simulink model "System_model"  (R2024b)
settings: Solver=ode1  StartTime=0.0  StopTime=12*3600  FixedStep=3600  RelTol=1e-3
values from neighbouring files (symbols this model uses):
  c = c_joule/3600    (= 1.16666666667)    [Dynamic.m]    (also in flat_plate_DHW.m = 4200)
  Ta = (Tmax+Tmin)/2 +(Tmax-Tmin)/2*cos(2*pi/24*(time_sun-tmax))    [Dynamic.m]    (also in flat_plate_DHW.m = (Ta_min+Ta_max)/2 + (-Ta_min+Ta_max)/2*cos(2*pi/24*(t-12)))
  time = (0:60*24)'    [Dynamic.m]
  Ts0 = out.Ts(end)    [parametric_analysis.m]
undefined symbols (not defined in the file or in its folder): dQd, dQr, hA, M
settings Model: Creator=giacm  LastModifiedBy=Andrea
settings DataIOCC: ReturnWorkspaceOutputs=off
settings RTWCC: GPUComputeCapability=3.5

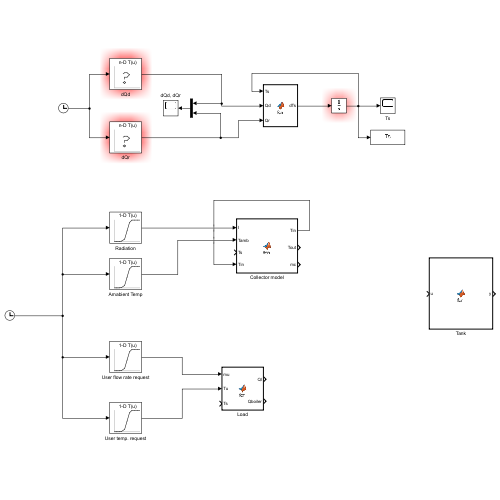
[thumbnail: Simulink's stored preview of the top-level diagram]
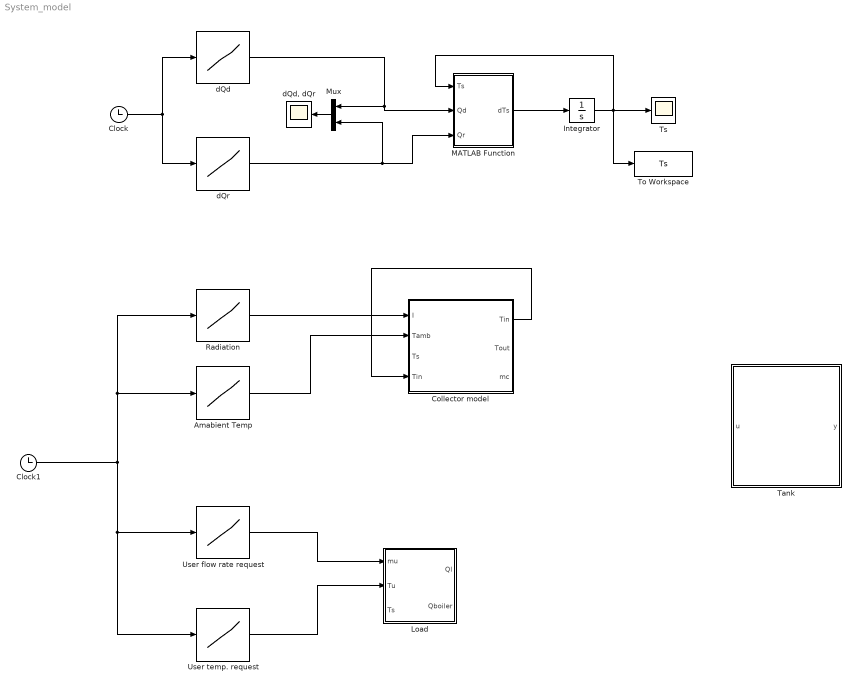
== system System_model ==
  Amabient Temp : Lookup_n-D  NumberOfTableDimensions=1  BreakpointsForDimension1=[-5:5]  Table=tanh([-5:5])  InternalRulePriority=Speed  RndMeth=Simplest
  Clock : Clock
  Clock1 : Clock
  Collector model : MATLAB Function  TreatAsAtomicUnit=on
  Integrator : Integrator  InitialCondition=Ts0
  Load : MATLAB Function  TreatAsAtomicUnit=on
  MATLAB Function : MATLAB Function  TreatAsAtomicUnit=on
  Mux : Mux  Inputs=2
  Radiation : Lookup_n-D  NumberOfTableDimensions=1  BreakpointsForDimension1=[-5:5]  Table=tanh([-5:5])  InternalRulePriority=Speed  RndMeth=Simplest
  Tank : MATLAB Function  TreatAsAtomicUnit=on
  To Workspace : ToWorkspace  VariableName=Ts  SaveFormat=Timeseries  SampleTime=-1
  Ts : Scope
  User flow rate request : Lookup_n-D  NumberOfTableDimensions=1  BreakpointsForDimension1=[-5:5]  Table=tanh([-5:5])  InternalRulePriority=Speed  RndMeth=Simplest
  User temp. request : Lookup_n-D  NumberOfTableDimensions=1  BreakpointsForDimension1=[-5:5]  Table=tanh([-5:5])  InternalRulePriority=Speed  RndMeth=Simplest
  dQd : Lookup_n-D  NumberOfTableDimensions=1  BreakpointsForDimension1=time  Table=dQd  InternalRulePriority=Speed  RndMeth=Simplest
  "dQd, dQr" : Scope
  dQr : Lookup_n-D  NumberOfTableDimensions=1  BreakpointsForDimension1=time  Table=dQr  InternalRulePriority=Speed  RndMeth=Simplest
  wires:
  MATLAB Function/1(dTs) -> Integrator/1
  Integrator/1 -> To Workspace/1, Ts/1, MATLAB Function/1(Ts)
  dQd/1 -> MATLAB Function/2(Qd), Mux/1
  dQr/1 -> Mux/2, MATLAB Function/3(Qr)
  Mux/1 -> "dQd, dQr"/1
  Clock/1 -> dQd/1, dQr/1
  Clock1/1 -> User flow rate request/1, User temp. request/1, Amabient Temp/1, Radiation/1
  Collector model/1(Tin) -> Collector model/4("Tin ")
  Amabient Temp/1 -> Collector model/2(Tamb)
  Radiation/1 -> Collector model/1(I)
  User flow rate request/1 -> Load/1(mu)
  User temp. request/1 -> Load/2(Tu)

== matlab function System_model/Collector model ==
  data: I input; Tamb input; Ts input; Tin output; Tout output; mc output; Tin input
function [Tin, Tout, mc] = fcn(I,Tamb,Ts, Tin)


%to add: starting from a set Tin, find a way to make eta calculate itself
eta = eta_zero - U * (Tin - Tamb) ./ I;

% Open valve only if we have irradiation and positive eta. Assume constant
% flow rate if valve is open (given by producer)

if(I > 0 && eta > 0)
    mc = m_dot;
else
    mc = 0;
end

collector_power = eta * I * A;

%wrong
%deltaT_collector = collector_power / (mc * c_joule)
%Tout = Tin + deltaT_collector;


%from Maple
Tout = (mc * c * effectiveness * Ts + collector_power) / (mc * c * effectiveness);
Tin = Tout - effectiveness * (Tout - Ts);

== matlab function System_model/MATLAB Function ==
  data: Ts input; dTs output; Qd input; Qr input; Ta parameter; hA parameter; M parameter; c parameter
function dTs = fcn(Ts,Qd,Qr,Ta, hA, M, c)

dTs = (Qd-Qr-hA*(Ts-Ta))/(M*c);

== matlab function System_model/Tank ==
  data: u input; y output
function y = fcn(u)

y = u;

== matlab function System_model/Load ==
  data: mu input; Ql output; Tu input; Ts input; Qboiler output
function [Ql, Qboiler] = fcn(mu, Tu, Ts)

if(Tu <= Ts)
    Ql = mu * c_joule * (Tu - Tmains);
else
    Ql = mu * c_joule * (Ts - Tmains);
end

if(Tu <= Ts)
    Qboiler = 0;
else
    Qboiler = mu * c_joule * (Tu - Ts);
end
